simulink model "process_dynamics_example"  (R2025a)
settings: Solver=FixedStepAuto  StartTime=0.0  StopTime=10.0  FixedStep=1e-3  RelTol=1e-3
libraries: simulink_extras x2, simulink x2
settings Model: Creator=mircea  LastModifiedBy=mircea

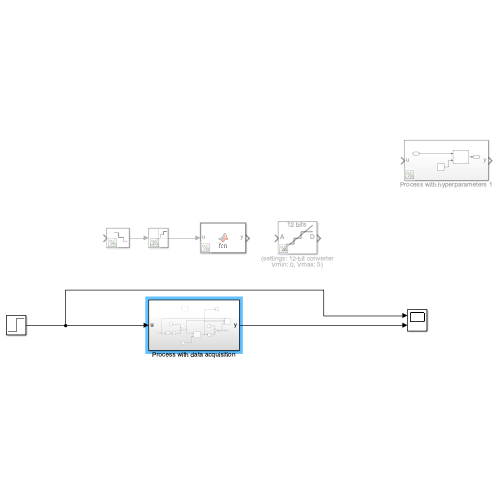
[thumbnail: Simulink's stored preview of the top-level diagram]
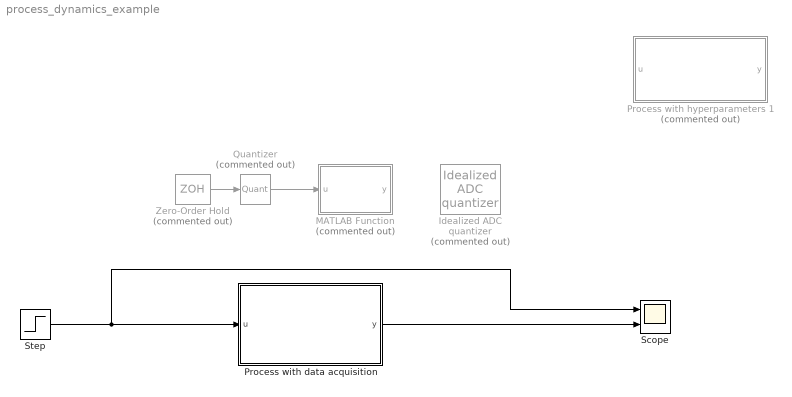
== system process_dynamics_example ==
  Idealized ADC quantizer : simulink_extras/Additional Discrete/Idealized ADC quantizer  Commented=on  NumberOfConverterBits=12  Vmin=0  Vmax=5  OutputDataType=int16  OutputNegativeValues=off
  MATLAB Function : MATLAB Function  Commented=on  TreatAsAtomicUnit=on
  Process with data acquisition : Subsystem
  Process with hyperparameters 1 : Subsystem  Commented=on
  Quantizer : Quantizer  Commented=on
  Scope : Scope  NumInputPorts=2
      settings: ActiveDisplayYMinimum=0.97954729585763611  ActiveDisplayYMaximum=1.0112520289648448
  Step : Step  SampleTime=0
  Zero-Order Hold : ZeroOrderHold  Commented=on  SampleTime=-1
  wires:
  Zero-Order Hold/1 -> Quantizer/1
  Quantizer/1 -> MATLAB Function/1(u)
  Step/1 -> Process with data acquisition/1(u), Scope/1
  Process with data acquisition/1(y) -> Scope/2

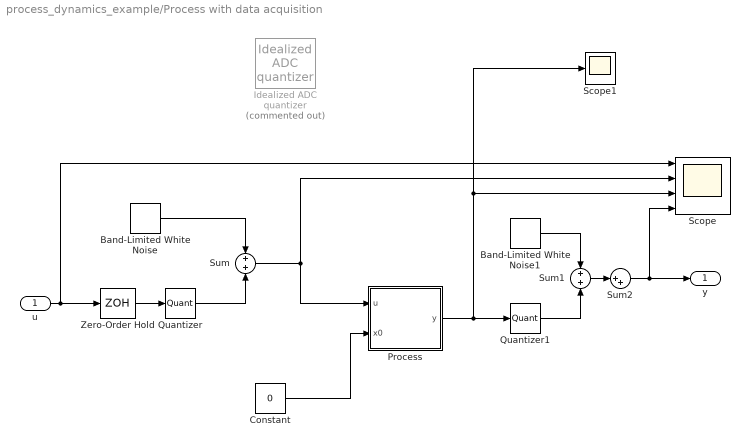
== system process_dynamics_example/Process with data acquisition ==
  u : Inport
  Band-Limited White Noise : simulink/Sources/Band-Limited White Noise  Cov=[1e-8]  Ts=1e-3  seed=[23341]
  Band-Limited White Noise1 : simulink/Sources/Band-Limited White Noise  Cov=[1e-8]  Ts=1e-3  seed=[23341]
  Constant : Constant  Value=0
  Idealized ADC quantizer : simulink_extras/Additional Discrete/Idealized ADC quantizer  Commented=on  NumberOfConverterBits=12  Vmin=-24  Vmax=24  OutputDataType=int16  OutputNegativeValues=off
  Process : Subsystem
  Quantizer : Quantizer  QuantizationInterval=9.7656e-04
  Quantizer1 : Quantizer  QuantizationInterval=9.7656e-04
  Scope : Scope  NumInputPorts=4
      settings: ActiveDisplayYMinimum=0.5972483393018001  ActiveDisplayYMaximum=0.98745694533475548
  Scope1 : Scope
      settings: ActiveDisplayYMinimum=-1  ActiveDisplayYMaximum=1  DataLoggingVariableName=ScopeData2
  Sum : Sum  Inputs=+|+
  Sum1 : Sum  Inputs=+|+
  Sum2 : Sum  Inputs=|++
  Zero-Order Hold : ZeroOrderHold  SampleTime=-1
  y : Outport
  wires:
  Process/1(y) -> Quantizer1/1, Scope1/1, Scope/3
  Constant/1 -> Process/2(x0)
  Band-Limited White Noise/1 -> Sum/1
  Sum/1 -> Scope/2, Process/1(u)
  Zero-Order Hold/1 -> Quantizer/1
  u/1 -> Scope/1, Zero-Order Hold/1
  Quantizer/1 -> Sum/2
  Band-Limited White Noise1/1 -> Sum1/1
  Quantizer1/1 -> Sum1/2
  Sum1/1 -> Sum2/1
  Sum2/1 -> Scope/4, y/1

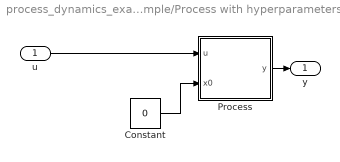
== system process_dynamics_example/Process with hyperparameters 1 ==
  u : Inport
  Constant : Constant  Value=0
  Process : Subsystem
  y : Outport
  wires:
  u/1 -> Process/1(u)
  Process/1(y) -> y/1
  Constant/1 -> Process/2(x0)

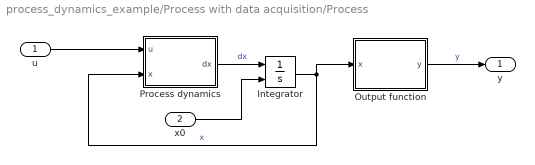
== system process_dynamics_example/Process with data acquisition/Process ==
  u : Inport
  x0 : Inport  Port=2
  Integrator : Integrator  InitialConditionSource=external
  Output function : MATLAB Function  TreatAsAtomicUnit=on
  Process dynamics : MATLAB Function  TreatAsAtomicUnit=on
  y : Outport
  wires:
  u/1 -> Process dynamics/1(u)
  Process dynamics/1(dx) -> Integrator/1  "dx"
  Integrator/1 -> Output function/1(x), Process dynamics/2(x)  "x"
  Output function/1(y) -> y/1  "y"
  x0/1 -> Integrator/2

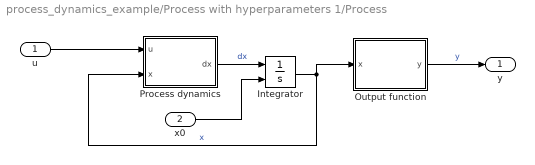
== system process_dynamics_example/Process with hyperparameters 1/Process ==
  u : Inport
  x0 : Inport  Port=2
  Integrator : Integrator  InitialConditionSource=external
  Output function : MATLAB Function  TreatAsAtomicUnit=on
  Process dynamics : MATLAB Function  TreatAsAtomicUnit=on
  y : Outport
  wires:
  u/1 -> Process dynamics/1(u)
  Process dynamics/1(dx) -> Integrator/1  "dx"
  Integrator/1 -> Output function/1(x), Process dynamics/2(x)  "x"
  Output function/1(y) -> y/1  "y"
  x0/1 -> Integrator/2

== matlab function process_dynamics_example/MATLAB Function ==
  data: u input; y output
function y = fcn(u)

y = u;

== matlab function process_dynamics_example/Process with data acquisition/Process/Output function ==
  data: y output; x input
function y = fcn(x)

y = x;

end

== matlab function process_dynamics_example/Process with hyperparameters 1/Process/Output function ==
  data: y output; x input
function y = fcn(x)

y = x;

end

== matlab function process_dynamics_example/Process with hyperparameters 1/Process/Process dynamics ==
  data: u input; dx output; x input
function dx = fcn(u,x)

dx = -x + u;

== matlab function process_dynamics_example/Process with data acquisition/Process/Process dynamics ==
  data: u input; dx output; x input
function dx = fcn(u,x)

dx = -x + u;
